simulink model "Sim_Runs_16p5"  (R2018b)
settings: Solver=FixedStepDiscrete  StartTime=0.0  StopTime=30  FixedStep=dt  RelTol=1e-3  EnableMultiTasking=on
PreLoadFcn:
  | DLLSimInit
InitFcn:
  | DLLSimInit
StartFcn:
  | tic
StopFcn:
  | SimTimeLaps = toc
values from neighbouring files (symbols this model uses):
  dt = 1/100    (= 0.01)    [DLLSimInit.m]    (also in DLLSimInit_SW.m; DLLSimInit_SW2.m; DLLSimInit_SW3.m)
  EngineLhFuelCut = 0    [DLLSimInit.m]    (also in DLLSimInit_SW.m; DLLSimInit_SW2.m; DLLSimInit_SW3.m)
  EngineRhFuelCut = 0    [DLLSimInit.m]    (also in DLLSimInit_SW.m; DLLSimInit_SW2.m; DLLSimInit_SW3.m)
  nDT = dt / SimDt    (= 6)    [DLLSimInit.m]    (also in DLLSimInit_SW.m; DLLSimInit_SW2.m; DLLSimInit_SW3.m)
  nOuputs = length(SaveList)    [DLLSimInit.m]    (also in DLLSimInit_SW.m; DLLSimInit_SW2.m; DLLSimInit_SW3.m)
  NWCastoring = 0    [DLLSimInit.m]
  PedalBrakeLh = 0    [DLLSimInit.m]    (also in DLLSimInit_SW.m; DLLSimInit_SW2.m; DLLSimInit_SW3.m)
  PedalBrakeRh = 0    [DLLSimInit.m]    (also in DLLSimInit_SW.m; DLLSimInit_SW2.m; DLLSimInit_SW3.m)
  RefWindDirDeg = WindDir    (= 90)    [DLLSimInit.m]    (also in DLLSimInit_SW.m; DLLSimInit_SW2.m; DLLSimInit_SW3.m)
  RefWindSpdKts = WindSpd    (= 0)    [DLLSimInit.m]    (also in DLLSimInit_SW.m; DLLSimInit_SW2.m; DLLSimInit_SW3.m)
  VertWindSpdKts = VertWindSpd    (= 0)    [DLLSimInit.m]
undefined symbols (not defined in the file or in its folder): DLLSimStep, sigbuilder_block, Trim_piccoloInCmd, Trim_REFSI_FD_IN_nmodeAftFlapCmd_Deg, Trim_REFSI_FD_IN_nmodeAilLhLowerCmd_Deg, Trim_REFSI_FD_IN_nmodeAilLhUpperCmd_Deg, Trim_REFSI_FD_IN_nmodeAilRhLowerCmd_Deg, Trim_REFSI_FD_IN_nmodeAilRhUpperCmd_Deg, Trim_REFSI_FD_IN_nmodeCgShifterCmd_Flag, Trim_REFSI_FD_IN_nmodeCgShifterCmd_Ft, Trim_REFSI_FD_IN_nmodeCgShifterNRCActive, Trim_REFSI_FD_IN_nmodeElvLhInbdCmd_Deg, Trim_REFSI_FD_IN_nmodeElvLhOutbdCmd_Deg, Trim_REFSI_FD_IN_nmodeElvLhUTailCmd_Deg, Trim_REFSI_FD_IN_nmodeElvRhInbdCmd_Deg, Trim_REFSI_FD_IN_nmodeElvRhOutbdCmd_Deg, Trim_REFSI_FD_IN_nmodeElvRhUTailCmd_Deg, Trim_REFSI_FD_IN_nmodeFlapLhIBCmd_Deg, Trim_REFSI_FD_IN_nmodeFlapLhOBCmd_Deg, Trim_REFSI_FD_IN_nmodeFlapRhIBCmd_Deg, Trim_REFSI_FD_IN_nmodeFlapRhOBCmd_Deg, Trim_REFSI_FD_IN_nmodeNoseGearCmd_Deg, Trim_REFSI_FD_IN_nmodeRudLhPylonCmd_Deg, Trim_REFSI_FD_IN_nmodeRudLhUTailCmd_Deg, Trim_REFSI_FD_IN_nmodeRudLhWingCmd_Deg, Trim_REFSI_FD_IN_nmodeRudRhPylonCmd_Deg, Trim_REFSI_FD_IN_nmodeRudRhUTailCmd_Deg, Trim_REFSI_FD_IN_nmodeRudRhWingCmd_Deg, Trim_REFSI_FD_IN_nmodeSlatLhCmd_Deg, Trim_REFSI_FD_IN_nmodeSlatRhCmd_Deg, Trim_REFSI_FD_IN_nmodeSplrLhInbdCmd_Deg, Trim_REFSI_FD_IN_nmodeSplrLhOutbdCmd_Deg, Trim_REFSI_FD_IN_nmodeSplrRhInbdCmd_Deg, Trim_REFSI_FD_IN_nmodeSplrRhOutbdCmd_Deg, Trim_REFSI_FD_IN_nmodeStabCmd, Trim_REFSI_FD_IN_nmodeTlaLhCmd_Deg, Trim_REFSI_FD_IN_nmodeTlaRhCmd_Deg
CloseFcn:
  | rtwprivate ssgencode ModelCloseRequest Sim_Runs
settings Model: ExtModeAutoUpdateStatusClock=off  Creator=b0514928  LastModifiedBy=B0532748
settings DataIOCC: LimitDataPoints=on  SaveFormat=Array  SaveState=on  SignalLogging=off
settings OptimizationCC: ExpressionDepthLimit=2147483647  LifeSpan=inf  SimCompilerOptimization=on
settings DebuggingCC: SaveWithParameterizedLinksMsg=none  UnderspecifiedInitializationDetection=Classic  MergeDetectMultiDrivingBlocksExec=none  SolverPrmCheckMsg=warning  StateNameClashWarn=warning  SFUnexpectedBacktrackingDiag=warning  SFNoUnconditionalDefaultTransitionDiag=warning  SFExecutionAtInitializationDiag=none
settings HardwareCC: ProdBitPerPointer=32  ProdBitPerSizeT=32  ProdBitPerPtrDiffT=32  ProdLargestAtomicFloat=None  ProdIntDivRoundTo=Undefined  ProdEndianess=Unspecified  ProdWordSize=32  ProdHWDeviceType=32-bit Generic
settings ModelReferenceCC: PropagateSignalLabelsOutOfModel=off
settings SFSimCC: SimUseLocalCustomCode=off
settings RTWCC: RTWUseLocalCustomCode=off
settings CodeAppCC: StateflowObjectComments=on
settings GRTTargetCC: TargetLangStandard=C89/C90 (ANSI)  GeneratePreprocessorConditionals=Disable all  CombineOutputUpdateFcns=off  GRTInterface=on
settings ConfigComp: CovMetricSettings=dw  CovHtmlReporting=on  CovSaveCumulativeToWorkspaceVar=on  CovSaveSingleToWorkspaceVar=on  CovExternalEMLEnable=off

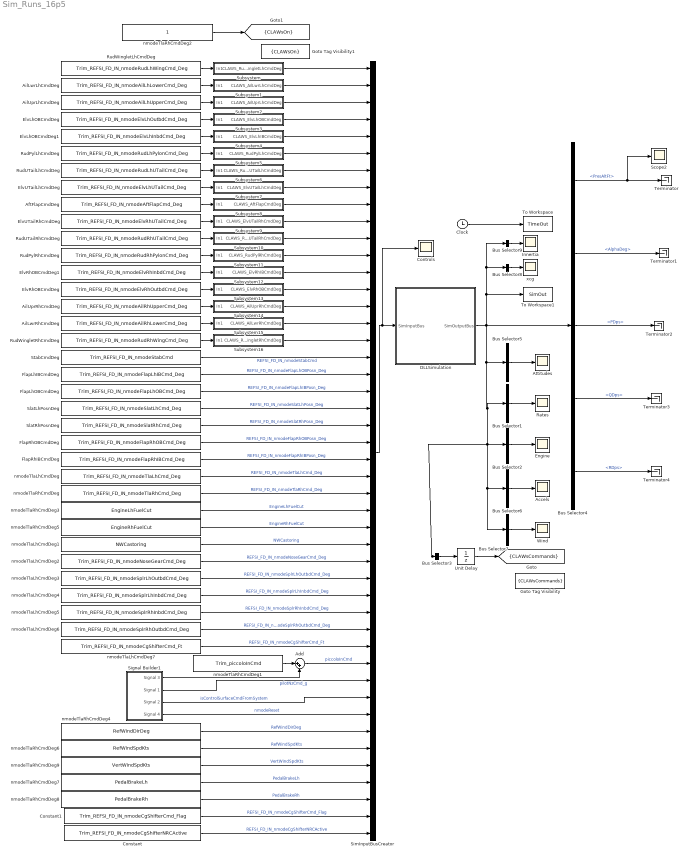
== system Sim_Runs_16p5 ==
  Accels : Scope
  Add : Sum  Inputs=|++
  AftFlapCmdDeg : Constant  Value=Trim_REFSI_FD_IN_nmodeAftFlapCmd_Deg
  AilLwrLhCmdDeg : Constant  Value=Trim_REFSI_FD_IN_nmodeAilLhLowerCmd_Deg
  AilLwrRhCmdDeg : Constant  Value=Trim_REFSI_FD_IN_nmodeAilRhLowerCmd_Deg
  AilUprLhCmdDeg : Constant  Value=Trim_REFSI_FD_IN_nmodeAilLhUpperCmd_Deg
  AilUprRhCmdDeg : Constant  Value=Trim_REFSI_FD_IN_nmodeAilRhUpperCmd_Deg
  Attitudes : Scope
  Bus Selector1 : BusSelector  OutputSignals=PDps,QDps,RDps  OutputAsBus=on
  Bus Selector2 : BusSelector  OutputSignals=XthrustLbs  OutputAsBus=on
  Bus Selector3 : BusSelector  OutputSignals=REFSI_AC_OUT_nmodeRudLhWingCmd_Deg,REFSI_AC_OUT_nmodeAilLhLowerCmd_Deg,REFSI_AC_OUT_nmodeAilLhUpperCmd_Deg,REFSI_AC_OUT_nmodeElvLhOutbdCmd_Deg,REFSI_AC_OUT_nmodeElvLhInbdCmd_Deg,REFSI_AC_OUT_nmodeRudLhPylonCmd_Deg,REFSI_AC_OUT_nmodeRudLhUTailCmd_Deg,REFSI_AC_OUT_nmodeElvLhUTailCmd_Deg,REFSI_AC_OUT_nmodeAftFlapCmd_Deg,REFSI_AC_OUT_nmodeElvRhUTailCmd_Deg,REFSI_AC_OUT_nmodeRudRhUTailCmd_Deg,REFSI_AC_OUT_nmodeRudRhPylonCmd_Deg,REFSI_AC_OUT_nmodeElvRhInbdCmd_Deg,REFSI_AC_OUT_nmodeElvRhOutbdCmd_Deg,REFSI_AC_OUT_nmodeAilRhUpperCmd_Deg,REFSI_AC_OUT_nmodeAilRhLowerCmd_Deg,REFSI_AC_OUT_nmodeRudRhWingCmd_Deg  OutputAsBus=on
  Bus Selector4 : BusSelector  OutputSignals=PresAltFt,AlphaDeg,PDps,QDps,RDps
  Bus Selector5 : BusSelector  OutputSignals=PhiDeg,ThetaDeg,PsiDeg  OutputAsBus=on
  Bus Selector6 : BusSelector  OutputSignals=NxG,NyG,NzG  OutputAsBus=on
  Bus Selector7 : BusSelector  OutputSignals=WindUFtps,WindVFtps,WindWFtps  OutputAsBus=on
  Bus Selector8 : BusSelector  OutputSignals=XcgPctMAC  OutputAsBus=on
  Bus Selector9 : BusSelector  OutputSignals=IxxLbsInch2,IyyLbsInch2,IzzLbsInch2,IxzLbsInch2  OutputAsBus=on
  Clock : Clock
  Constant : Constant  Value=Trim_REFSI_FD_IN_nmodeCgShifterNRCActive
  Constant1 : Constant  Value=Trim_REFSI_FD_IN_nmodeCgShifterCmd_Flag
  Controls : Scope
  DLLSimulation : Subsystem
  ElvLhOBCmdDeg : Constant  Value=Trim_REFSI_FD_IN_nmodeElvLhOutbdCmd_Deg
  ElvLhOBCmdDeg1 : Constant  Value=Trim_REFSI_FD_IN_nmodeElvLhInbdCmd_Deg
  ElvRhOBCmdDeg : Constant  Value=Trim_REFSI_FD_IN_nmodeElvRhOutbdCmd_Deg
  ElvRhOBCmdDeg1 : Constant  Value=Trim_REFSI_FD_IN_nmodeElvRhInbdCmd_Deg
  ElvUTailLhCmdDeg : Constant  Value=Trim_REFSI_FD_IN_nmodeElvLhUTailCmd_Deg
  ElvUTailRhCmdDeg : Constant  Value=Trim_REFSI_FD_IN_nmodeElvRhUTailCmd_Deg
  Engine : Scope
  FlapLhIBCmdDeg : Constant  Value=Trim_REFSI_FD_IN_nmodeFlapLhIBCmd_Deg
  FlapLhOBCmdDeg : Constant  Value=Trim_REFSI_FD_IN_nmodeFlapLhOBCmd_Deg
  FlapRhIBCmdDeg : Constant  Value=Trim_REFSI_FD_IN_nmodeFlapRhIBCmd_Deg
  FlapRhOBCmdDeg : Constant  Value=Trim_REFSI_FD_IN_nmodeFlapRhOBCmd_Deg
  Goto Tag Visibility : GotoTagVisibility  GotoTag=CLAWsCommands
  Goto Tag Visibility1 : GotoTagVisibility  GotoTag=CLAWsOn
  Innertia : Scope
  Rates : Scope
  RudPylLhCmdDeg : Constant  Value=Trim_REFSI_FD_IN_nmodeRudLhPylonCmd_Deg
  RudPylRhCmdDeg : Constant  Value=Trim_REFSI_FD_IN_nmodeRudRhPylonCmd_Deg
  RudUTailLhCmdDeg : Constant  Value=Trim_REFSI_FD_IN_nmodeRudLhUTailCmd_Deg
  RudUTailRhCmdDeg : Constant  Value=Trim_REFSI_FD_IN_nmodeRudRhUTailCmd_Deg
  RudWingletLhCmdDeg : Constant  Value=Trim_REFSI_FD_IN_nmodeRudLhWingCmd_Deg
  RudWingletRhCmdDeg : Constant  Value=Trim_REFSI_FD_IN_nmodeRudRhWingCmd_Deg
  Scope2 : Scope
  Signal Builder1 : Subsystem  Tag=STV Subsys  LoadFcn=sigbuilder_block('load');  StartFcn=sigbuilder_block('start');  StopFcn=sigbuilder_block('stop');  ClipboardFcn=sigbuilder_block('clipboard');  mask(Sigbuilder block){tuvar=[0:10]}
      mask help: Simulink:masks:SigbuilderBlock_MD
      mask init:
      | if ~strcmp(get_param(bdroot(gcbh),'SimulationStatus'),'stopped') tuvar = sigbuilder_block('maskInit'); end
      settings: CopyFcn=sigbuilder_block('copy');  DeleteFcn=sigbuilder_block('delete');  ModelCloseFcn=sigbuilder_block('modelClose');  PreSaveFcn=sigbuilder_block('preSave');  PauseFcn=sigbuilder_block('pause');  ContinueFcn=sigbuilder_block('continue');  NameChangeFcn=sigbuilder_block('namechange');  OpenFcn=sigbuilder_block('open',[703.5 198.75 550.5 360 ]);  CloseFcn=sigbuilder_block('close');
      mask Display: plot(0, 0, 100, 100,[2, 2, 32, 32, 2], [68, 8, 8, 68, 68],[32, 2], [38, 38], [32, 19, 2],[53, 60, 44], [32, 17, 17, 2],[16, 16, 31, 31]);txt = getActiveGroup(gcbh);text(2, 100, txt,'verticalAlignment', 'top');
  SimInputBusCreator : BusCreator  Inputs=46
  SlatLhPosnDeg : Constant  Value=Trim_REFSI_FD_IN_nmodeSlatLhCmd_Deg
  SlatRhPosnDeg : Constant  Value=Trim_REFSI_FD_IN_nmodeSlatRhCmd_Deg
  StabCmdDeg : Constant  Value=Trim_REFSI_FD_IN_nmodeStabCmd
  Subsystem : Subsystem
  Subsystem1 : Subsystem
  Subsystem10 : Subsystem
  Subsystem11 : Subsystem
  Subsystem12 : Subsystem
  Subsystem13 : Subsystem
  Subsystem14 : Subsystem
  Subsystem15 : Subsystem
  Subsystem16 : Subsystem
  Subsystem2 : Subsystem
  Subsystem3 : Subsystem
  Subsystem4 : Subsystem
  Subsystem5 : Subsystem
  Subsystem6 : Subsystem
  Subsystem7 : Subsystem
  Subsystem8 : Subsystem
  Subsystem9 : Subsystem
  Terminator{,1..4} (5 alike) : Terminator
  To Workspace : ToWorkspace  VariableName=TimeOut  SaveFormat=Structure With Time  SampleTime=-1
  To Workspace1 : ToWorkspace  VariableName=SimOut  SaveFormat=Structure With Time  SampleTime=-1
  Unit Delay : UnitDelay  SampleTime=-1
  Wind : Scope
  nmodeTlaLhCmdDeg : Constant  Value=Trim_REFSI_FD_IN_nmodeTlaLhCmd_Deg
  nmodeTlaLhCmdDeg1 : Constant  Value=NWCastoring
  nmodeTlaLhCmdDeg2 : Constant  Value=Trim_REFSI_FD_IN_nmodeNoseGearCmd_Deg
  nmodeTlaLhCmdDeg3 : Constant  Value=Trim_REFSI_FD_IN_nmodeSplrLhOutbdCmd_Deg
  nmodeTlaLhCmdDeg4 : Constant  Value=Trim_REFSI_FD_IN_nmodeSplrLhInbdCmd_Deg
  nmodeTlaLhCmdDeg5 : Constant  Value=Trim_REFSI_FD_IN_nmodeSplrRhInbdCmd_Deg
  nmodeTlaLhCmdDeg6 : Constant  Value=Trim_REFSI_FD_IN_nmodeSplrRhOutbdCmd_Deg
  nmodeTlaLhCmdDeg7 : Constant  Value=Trim_REFSI_FD_IN_nmodeCgShifterCmd_Ft
  nmodeTlaRhCmdDeg : Constant  Value=Trim_REFSI_FD_IN_nmodeTlaRhCmd_Deg
  nmodeTlaRhCmdDeg1 : Constant  Value=Trim_piccoloInCmd
  nmodeTlaRhCmdDeg2 : Constant
  nmodeTlaRhCmdDeg3 : Constant  Value=EngineLhFuelCut
  nmodeTlaRhCmdDeg4 : Constant  Value=RefWindDirDeg
  nmodeTlaRhCmdDeg5 : Constant  Value=EngineRhFuelCut
  nmodeTlaRhCmdDeg6 : Constant  Value=RefWindSpdKts
  nmodeTlaRhCmdDeg7 : Constant  Value=PedalBrakeLh
  nmodeTlaRhCmdDeg8 : Constant  Value=PedalBrakeRh
  nmodeTlaRhCmdDeg9 : Constant  Value=VertWindSpdKts
  xcg : Scope
  tag scope: CLAWsCommands=scoped, CLAWsOn=scoped
  wires:
  Clock/1 -> To Workspace/1
  SimInputBusCreator/1 -> Controls/1, DLLSimulation/1(SimInputBus)
  Bus Selector4/1 -> Scope2/1, Terminator/1  "<PresAltFt>"
  Bus Selector4/2 -> Terminator1/1  "<AlphaDeg>"
  Bus Selector4/3 -> Terminator2/1  "<PDps>"
  Bus Selector4/4 -> Terminator3/1  "<QDps>"
  Bus Selector4/5 -> Terminator4/1  "<RDps>"
  AilLwrLhCmdDeg/1 -> Subsystem1/1(In1)
  AilUprLhCmdDeg/1 -> Subsystem2/1(In1)
  ElvLhOBCmdDeg/1 -> Subsystem3/1(In1)
  RudPylLhCmdDeg/1 -> Subsystem5/1(In1)
  RudUTailLhCmdDeg/1 -> Subsystem6/1(In1)
  ElvUTailLhCmdDeg/1 -> Subsystem7/1(In1)
  AftFlapCmdDeg/1 -> Subsystem8/1(In1)
  ElvUTailRhCmdDeg/1 -> Subsystem9/1(In1)
  RudUTailRhCmdDeg/1 -> Subsystem10/1(In1)
  RudPylRhCmdDeg/1 -> Subsystem11/1(In1)
  ElvRhOBCmdDeg/1 -> Subsystem13/1(In1)
  AilUprRhCmdDeg/1 -> Subsystem14/1(In1)
  AilLwrRhCmdDeg/1 -> Subsystem15/1(In1)
  RudWingletRhCmdDeg/1 -> Subsystem16/1(In1)
  StabCmdDeg/1 -> SimInputBusCreator/18  "REFSI_FD_IN_nmodeStabCmd"
  FlapLhIBCmdDeg/1 -> SimInputBusCreator/19  "REFSI_FD_IN_nmodeFlapLhOBPosn_Deg"
  FlapLhOBCmdDeg/1 -> SimInputBusCreator/20  "REFSI_FD_IN_nmodeFlapLhIBPosn_Deg"
  SlatLhPosnDeg/1 -> SimInputBusCreator/21  "REFSI_FD_IN_nmodeSlatLhPosn_Deg"
  SlatRhPosnDeg/1 -> SimInputBusCreator/22  "REFSI_FD_IN_nmodeSlatRhPosn_Deg"
  FlapRhOBCmdDeg/1 -> SimInputBusCreator/23  "REFSI_FD_IN_nmodeFlapRhOBPosn_Deg"
  FlapRhIBCmdDeg/1 -> SimInputBusCreator/24  "REFSI_FD_IN_nmodeFlapRhIBPosn_Deg"
  nmodeTlaLhCmdDeg/1 -> SimInputBusCreator/25  "REFSI_FD_IN_nmodeTlaLhCmd_Deg"
  nmodeTlaRhCmdDeg/1 -> SimInputBusCreator/26  "REFSI_FD_IN_nmodeTlaRhCmd_Deg"
  Bus Selector2/1 -> Engine/1
  Bus Selector1/1 -> Rates/1
  DLLSimulation/1(SimOutputBus) -> Bus Selector4/1, Bus Selector9/1, Bus Selector8/1, To Workspace1/1, Bus Selector5/1, Bus Selector7/1, Bus Selector6/1, Bus Selector3/1, Bus Selector2/1, Bus Selector1/1
  ElvLhOBCmdDeg1/1 -> Subsystem4/1(In1)
  ElvRhOBCmdDeg1/1 -> Subsystem12/1(In1)
  Bus Selector3/1 -> Unit Delay/1
  RudWingletLhCmdDeg/1 -> Subsystem/1(In1)
  Subsystem/1(CLAWS_RudWingletLhCmdDeg) -> SimInputBusCreator/1
  Subsystem1/1(CLAWS_AilLwrLhCmdDeg) -> SimInputBusCreator/2
  Subsystem2/1(CLAWS_AilUprLhCmdDeg) -> SimInputBusCreator/3
  Subsystem3/1(CLAWS_ElvLhOBCmdDeg) -> SimInputBusCreator/4
  Subsystem4/1(CLAWS_ElvLhIBCmdDeg) -> SimInputBusCreator/5
  Subsystem5/1(CLAWS_RudPylLhCmdDeg) -> SimInputBusCreator/6
  Subsystem6/1(CLAWS_RudUTailLhCmdDeg) -> SimInputBusCreator/7
  Subsystem7/1(CLAWS_ElvUTailLhCmdDeg) -> SimInputBusCreator/8
  Subsystem8/1(CLAWS_AftFlapCmdDeg) -> SimInputBusCreator/9
  Subsystem9/1(CLAWS_ElvUTailRhCmdDeg) -> SimInputBusCreator/10
  Subsystem10/1(CLAWS_RudUTailRhCmdDeg) -> SimInputBusCreator/11
  Subsystem11/1(CLAWS_RudPylRhCmdDeg) -> SimInputBusCreator/12
  Subsystem12/1(CLAWS_ElvRhIBCmdDeg) -> SimInputBusCreator/13
  Subsystem13/1(CLAWS_ElvRhOBCmdDeg) -> SimInputBusCreator/14
  Subsystem14/1(CLAWS_AilUprRhCmdDeg) -> SimInputBusCreator/15
  Subsystem15/1(CLAWS_AilLwrRhCmdDeg) -> SimInputBusCreator/16
  Subsystem16/1(CLAWS_RudWingletRhCmdDeg) -> SimInputBusCreator/17
  nmodeTlaRhCmdDeg2/1 -> [CLAWsOn]
  Unit Delay/1 -> [CLAWsCommands]
  nmodeTlaRhCmdDeg1/1 -> Add/1
  Add/1 -> SimInputBusCreator/36  "piccoloInCmd"
  Signal Builder1/1(Signal 3) -> Add/2
  Signal Builder1/2(Signal 1) -> SimInputBusCreator/37  "pilotNzCmd_g"
  Signal Builder1/3(Signal 2) -> SimInputBusCreator/38  "isControlSurfaceCmdFromSystem"
  Signal Builder1/4(Signal 4) -> SimInputBusCreator/39  "nmodeReset"
  Bus Selector5/1 -> Attitudes/1
  Bus Selector6/1 -> Accels/1
  nmodeTlaLhCmdDeg2/1 -> SimInputBusCreator/30  "REFSI_FD_IN_nmodeNoseGearCmd_Deg"
  Bus Selector8/1 -> xcg/1
  Bus Selector9/1 -> Innertia/1
  Bus Selector7/1 -> Wind/1
  nmodeTlaLhCmdDeg3/1 -> SimInputBusCreator/31  "REFSI_FD_IN_nmodeSplrLhOutbdCmd_Deg"
  nmodeTlaLhCmdDeg4/1 -> SimInputBusCreator/32  "REFSI_FD_IN_nmodeSplrLhInbdCmd_Deg"
  nmodeTlaLhCmdDeg5/1 -> SimInputBusCreator/33  "REFSI_FD_IN_nmodeSplrRhInbdCmd_Deg"
  nmodeTlaLhCmdDeg6/1 -> SimInputBusCreator/34  "REFSI_FD_IN_nmodeSplrRhOutbdCmd_Deg"
  nmodeTlaLhCmdDeg7/1 -> SimInputBusCreator/35  "REFSI_FD_IN_nmodeCgShifterCmd_Ft"
  nmodeTlaLhCmdDeg1/1 -> SimInputBusCreator/29  "NWCastoring"
  nmodeTlaRhCmdDeg3/1 -> SimInputBusCreator/27  "EngineLhFuelCut"
  nmodeTlaRhCmdDeg5/1 -> SimInputBusCreator/28  "EngineRhFuelCut"
  nmodeTlaRhCmdDeg4/1 -> SimInputBusCreator/40  "RefWindDirDeg"
  nmodeTlaRhCmdDeg6/1 -> SimInputBusCreator/41  "RefWindSpdKts"
  nmodeTlaRhCmdDeg7/1 -> SimInputBusCreator/43  "PedalBrakeLh"
  nmodeTlaRhCmdDeg8/1 -> SimInputBusCreator/44  "PedalBrakeRh"
  nmodeTlaRhCmdDeg9/1 -> SimInputBusCreator/42  "VertWindSpdKts"
  Constant1/1 -> SimInputBusCreator/45  "REFSI_FD_IN_nmodeCgShifterCmd_Flag"
  Constant/1 -> SimInputBusCreator/46  "REFSI_FD_IN_nmodeCgShifterNRCActive"

== system Sim_Runs_16p5/DLLSimulation ==
  SimInputBus : Inport
  Bus2Vect2 : Subsystem
      mask init:
      | CurrentSys = gcs;
      | blockName = get_param(gcb,'Name');
      | 
      | CurBlk = [CurrentSys,'/',blockName];%Current block
      | BusSel = [CurrentSys,'/',blockName,'/BusSelector'];%BusSelectorBlock
      | BusMux = [CurrentSys,'/',blockName,'/Mux'];%Mux bloxk
      | 
      | 
      | 
      | Inputs = get_param(BusSel,'InputSignals');
      | 
      | 
      | outsig='';
      | for i=1:length(Inputs)
      |     outsig=[outsig Inputs{i} ','];
      | end;
      | outsig=outsig(1:length(outsig)-1);
      | 
      |     for nnn = 1:str2double(get_param(BusMux,'Inputs'))
      |         delete_line([CurrentSys '/' blockName],['BusSelector/' num2str(nnn)],['Mux/' num2str(nnn)])
      |     end
      |     
      | set_param(BusSel,'OutputSignals',outsig);
      | set_param(BusMux,'Inputs',num2str(length(Inputs)))
      | 
      | 
      | 
      |     
      |     for nnn = 1:length(Inputs)
      |         add_line([CurrentSys '/' blockName],['BusSelector/' num2str(nnn)],['Mux/' num2str(nnn)])
      |     end
  DLLSimulationStep : MATLABFcn  MATLABFcn=DLLSimStep(u,nDT)  OutputDimensions=nOuputs  SampleTime=dt
  Vector to Bus : Subsystem  mask{Nsigs=nOuputs}
      mask prompts: Nsigs "Signal Length"
  SimOutputBus : Outport
  wires:
  Bus2Vect2/1(Out1) -> DLLSimulationStep/1
  DLLSimulationStep/1 -> Vector to Bus/1(In1)
  Vector to Bus/1(Out1) -> SimOutputBus/1
  SimInputBus/1 -> Bus2Vect2/1(In1)

== system Sim_Runs_16p5/Signal Builder1 ==
  Demux : Demux  Tag=STV Demux
  FromWs : FromWorkspace  Tag=STV FromWs  VariableName=tuvar  SampleTime=0
      SigBuilderData=|
      | common.afterFinalStr = 'Extrapolate'
      | common.sampleTime = 0
      | dataSet.timeRange = [0 50]
      | dataSet.name = 'Group 1'
      | sbobj.Groups.Name = 'Group 1'
      | sbobj.Groups.Signals(1).Name = 'Signal 3'
      | sbobj.Groups.Signals(1).XData = [0 1 1 50]
      | sbobj.Groups.Signals(1).YData = [0 0 -1 -1]
      | sbobj.Groups.Signals(2).Name = 'Signal 1'
      | sbobj.Groups.Signals(2).XData = [0 20 20 30 30 50]
      | sbobj.Groups.Signals(2).YData = [0 0 0.4 0.4 0 0]
      | sbobj.Groups.Signals(3).Name = 'Signal 2'
      | sbobj.Groups.Signals(3).XData = [0 0.5 0.5 50]
      | sbobj.Groups.Signals(3).YData = [1 1 0 0]
      | sbobj.Groups.Signals(4).Name = 'Signal 4'
      | sbobj.Groups.Signals(4).XData = [0 0.1 0.1 50]
      | sbobj.Groups.Signals(4).YData = [1 1 0 0]
      | sbobj.Groups.TimeRange = [0 50]
  Signal 3 : Outport  Tag=STV Outport
  Signal 1 : Outport  Tag=STV Outport  Port=2
  Signal 2 : Outport  Tag=STV Outport  Port=3
  Signal 4 : Outport  Tag=STV Outport  Port=4
  wires:
  FromWs/1 -> Demux/1
  Demux/1 -> Signal 3/1
  Demux/2 -> Signal 1/1
  Demux/3 -> Signal 2/1
  Demux/4 -> Signal 4/1

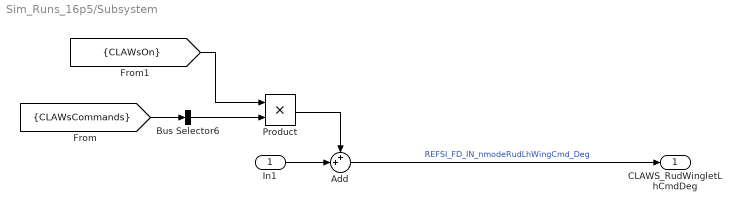
== system Sim_Runs_16p5/Subsystem ==
  In1 : Inport
  Add : Sum  Inputs=++|
  Bus Selector6 : BusSelector  OutputSignals=REFSI_AC_OUT_nmodeRudLhWingCmd_Deg  OutputAsBus=on
  Product : Product
  CLAWS_RudWingletLhCmdDeg : Outport
  wires:
  Add/1 -> CLAWS_RudWingletLhCmdDeg/1  "REFSI_FD_IN_nmodeRudLhWingCmd_Deg"
  [CLAWsCommands] -> Bus Selector6/1
  In1/1 -> Add/2
  Bus Selector6/1 -> Product/2
  Product/1 -> Add/1
  [CLAWsOn] -> Product/1

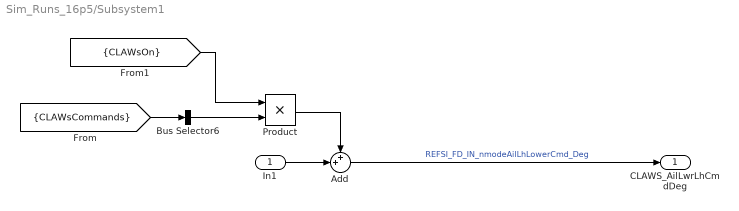
== system Sim_Runs_16p5/Subsystem1 ==
  In1 : Inport
  Add : Sum  Inputs=++|
  Bus Selector6 : BusSelector  OutputSignals=REFSI_AC_OUT_nmodeAilLhLowerCmd_Deg  OutputAsBus=on
  Product : Product
  CLAWS_AilLwrLhCmdDeg : Outport
  wires:
  [CLAWsOn] -> Product/1
  Product/1 -> Add/1
  Bus Selector6/1 -> Product/2
  In1/1 -> Add/2
  [CLAWsCommands] -> Bus Selector6/1
  Add/1 -> CLAWS_AilLwrLhCmdDeg/1  "REFSI_FD_IN_nmodeAilLhLowerCmd_Deg"

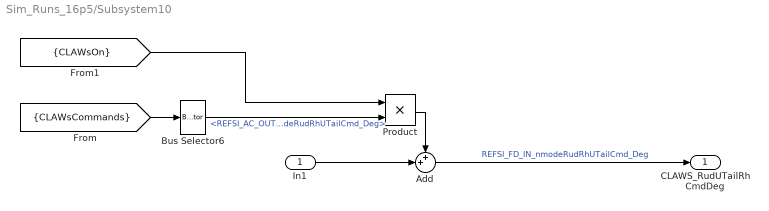
== system Sim_Runs_16p5/Subsystem10 ==
  In1 : Inport
  Add : Sum  Inputs=++|
  Bus Selector6 : BusSelector  OutputSignals=REFSI_AC_OUT_nmodeRudRhUTailCmd_Deg
  Product : Product
  CLAWS_RudUTailRhCmdDeg : Outport
  wires:
  Add/1 -> CLAWS_RudUTailRhCmdDeg/1  "REFSI_FD_IN_nmodeRudRhUTailCmd_Deg"
  [CLAWsCommands] -> Bus Selector6/1
  In1/1 -> Add/2
  Bus Selector6/1 -> Product/2  "<REFSI_AC_OUT_nmodeRudRhUTailCmd_Deg>"
  Product/1 -> Add/1
  [CLAWsOn] -> Product/1

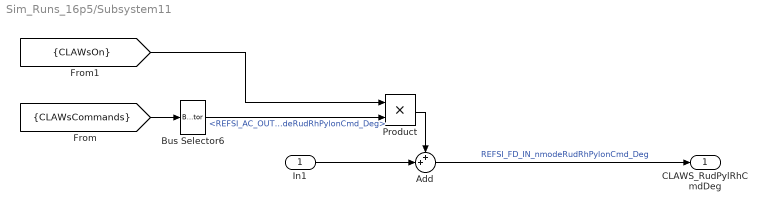
== system Sim_Runs_16p5/Subsystem11 ==
  In1 : Inport
  Add : Sum  Inputs=++|
  Bus Selector6 : BusSelector  OutputSignals=REFSI_AC_OUT_nmodeRudRhPylonCmd_Deg
  Product : Product
  CLAWS_RudPylRhCmdDeg : Outport
  wires:
  [CLAWsOn] -> Product/1
  Product/1 -> Add/1
  Bus Selector6/1 -> Product/2  "<REFSI_AC_OUT_nmodeRudRhPylonCmd_Deg>"
  In1/1 -> Add/2
  [CLAWsCommands] -> Bus Selector6/1
  Add/1 -> CLAWS_RudPylRhCmdDeg/1  "REFSI_FD_IN_nmodeRudRhPylonCmd_Deg"

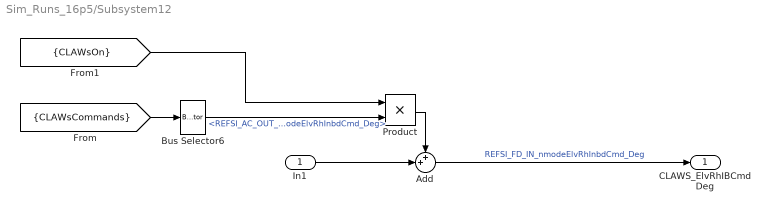
== system Sim_Runs_16p5/Subsystem12 ==
  In1 : Inport
  Add : Sum  Inputs=++|
  Bus Selector6 : BusSelector  OutputSignals=REFSI_AC_OUT_nmodeElvRhInbdCmd_Deg
  Product : Product
  CLAWS_ElvRhIBCmdDeg : Outport
  wires:
  Add/1 -> CLAWS_ElvRhIBCmdDeg/1  "REFSI_FD_IN_nmodeElvRhInbdCmd_Deg"
  [CLAWsCommands] -> Bus Selector6/1
  In1/1 -> Add/2
  Bus Selector6/1 -> Product/2  "<REFSI_AC_OUT_nmodeElvRhInbdCmd_Deg>"
  Product/1 -> Add/1
  [CLAWsOn] -> Product/1

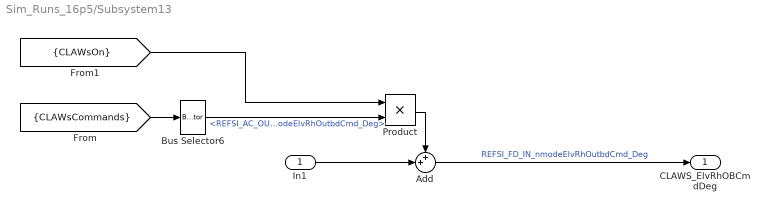
== system Sim_Runs_16p5/Subsystem13 ==
  In1 : Inport
  Add : Sum  Inputs=++|
  Bus Selector6 : BusSelector  OutputSignals=REFSI_AC_OUT_nmodeElvRhOutbdCmd_Deg
  Product : Product
  CLAWS_ElvRhOBCmdDeg : Outport
  wires:
  [CLAWsOn] -> Product/1
  Product/1 -> Add/1
  Bus Selector6/1 -> Product/2  "<REFSI_AC_OUT_nmodeElvRhOutbdCmd_Deg>"
  In1/1 -> Add/2
  [CLAWsCommands] -> Bus Selector6/1
  Add/1 -> CLAWS_ElvRhOBCmdDeg/1  "REFSI_FD_IN_nmodeElvRhOutbdCmd_Deg"

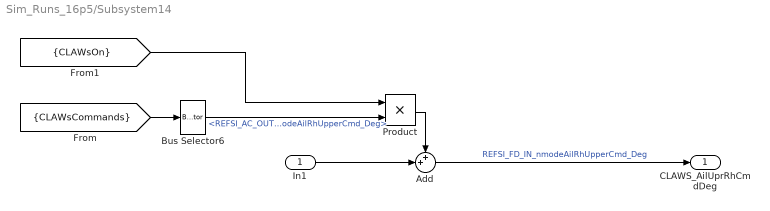
== system Sim_Runs_16p5/Subsystem14 ==
  In1 : Inport
  Add : Sum  Inputs=++|
  Bus Selector6 : BusSelector  OutputSignals=REFSI_AC_OUT_nmodeAilRhUpperCmd_Deg
  Product : Product
  CLAWS_AilUprRhCmdDeg : Outport
  wires:
  Add/1 -> CLAWS_AilUprRhCmdDeg/1  "REFSI_FD_IN_nmodeAilRhUpperCmd_Deg"
  [CLAWsCommands] -> Bus Selector6/1
  In1/1 -> Add/2
  Bus Selector6/1 -> Product/2  "<REFSI_AC_OUT_nmodeAilRhUpperCmd_Deg>"
  Product/1 -> Add/1
  [CLAWsOn] -> Product/1

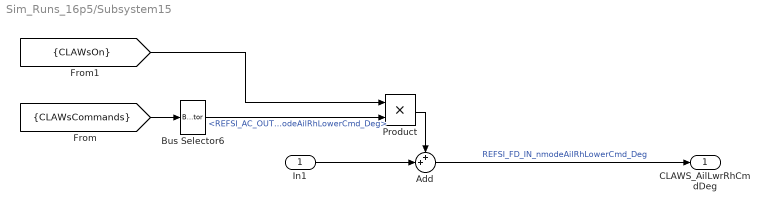
== system Sim_Runs_16p5/Subsystem15 ==
  In1 : Inport
  Add : Sum  Inputs=++|
  Bus Selector6 : BusSelector  OutputSignals=REFSI_AC_OUT_nmodeAilRhLowerCmd_Deg
  Product : Product
  CLAWS_AilLwrRhCmdDeg : Outport
  wires:
  [CLAWsOn] -> Product/1
  Product/1 -> Add/1
  Bus Selector6/1 -> Product/2  "<REFSI_AC_OUT_nmodeAilRhLowerCmd_Deg>"
  In1/1 -> Add/2
  [CLAWsCommands] -> Bus Selector6/1
  Add/1 -> CLAWS_AilLwrRhCmdDeg/1  "REFSI_FD_IN_nmodeAilRhLowerCmd_Deg"

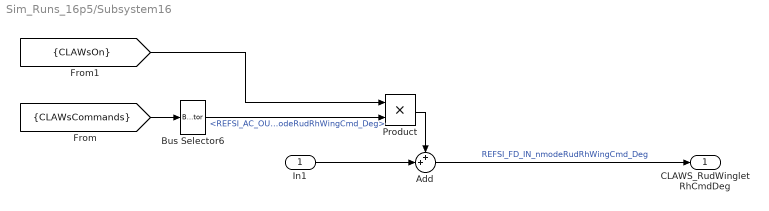
== system Sim_Runs_16p5/Subsystem16 ==
  In1 : Inport
  Add : Sum  Inputs=++|
  Bus Selector6 : BusSelector  OutputSignals=REFSI_AC_OUT_nmodeRudRhWingCmd_Deg
  Product : Product
  CLAWS_RudWingletRhCmdDeg : Outport
  wires:
  Add/1 -> CLAWS_RudWingletRhCmdDeg/1  "REFSI_FD_IN_nmodeRudRhWingCmd_Deg"
  [CLAWsCommands] -> Bus Selector6/1
  In1/1 -> Add/2
  Bus Selector6/1 -> Product/2  "<REFSI_AC_OUT_nmodeRudRhWingCmd_Deg>"
  Product/1 -> Add/1
  [CLAWsOn] -> Product/1

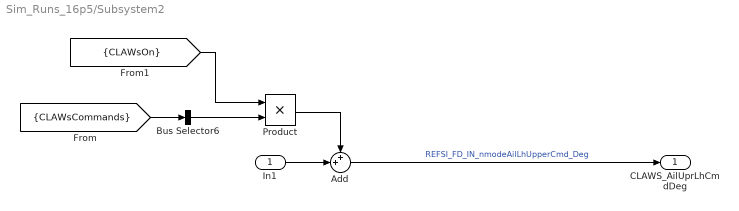
== system Sim_Runs_16p5/Subsystem2 ==
  In1 : Inport
  Add : Sum  Inputs=++|
  Bus Selector6 : BusSelector  OutputSignals=REFSI_AC_OUT_nmodeAilLhUpperCmd_Deg  OutputAsBus=on
  Product : Product
  CLAWS_AilUprLhCmdDeg : Outport
  wires:
  Add/1 -> CLAWS_AilUprLhCmdDeg/1  "REFSI_FD_IN_nmodeAilLhUpperCmd_Deg"
  [CLAWsCommands] -> Bus Selector6/1
  In1/1 -> Add/2
  Bus Selector6/1 -> Product/2
  Product/1 -> Add/1
  [CLAWsOn] -> Product/1

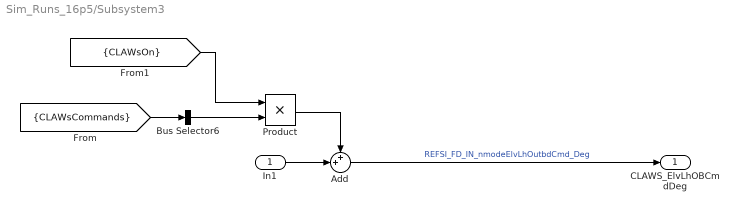
== system Sim_Runs_16p5/Subsystem3 ==
  In1 : Inport
  Add : Sum  Inputs=++|
  Bus Selector6 : BusSelector  OutputSignals=REFSI_AC_OUT_nmodeElvLhOutbdCmd_Deg  OutputAsBus=on
  Product : Product
  CLAWS_ElvLhOBCmdDeg : Outport
  wires:
  [CLAWsOn] -> Product/1
  Product/1 -> Add/1
  Bus Selector6/1 -> Product/2
  In1/1 -> Add/2
  [CLAWsCommands] -> Bus Selector6/1
  Add/1 -> CLAWS_ElvLhOBCmdDeg/1  "REFSI_FD_IN_nmodeElvLhOutbdCmd_Deg"

== system Sim_Runs_16p5/Subsystem4 ==
  In1 : Inport
  Add : Sum  Inputs=++|
  Bus Selector6 : BusSelector  OutputSignals=REFSI_AC_OUT_nmodeElvLhInbdCmd_Deg  OutputAsBus=on
  Product : Product
  CLAWS_ElvLhIBCmdDeg : Outport
  wires:
  Add/1 -> CLAWS_ElvLhIBCmdDeg/1  "REFSI_FD_IN_nmodeElvLhInbdCmd_Deg"
  [CLAWsCommands] -> Bus Selector6/1
  In1/1 -> Add/2
  Bus Selector6/1 -> Product/2
  Product/1 -> Add/1
  [CLAWsOn] -> Product/1

== system Sim_Runs_16p5/Subsystem5 ==
  In1 : Inport
  Add : Sum  Inputs=++|
  Bus Selector6 : BusSelector  OutputSignals=REFSI_AC_OUT_nmodeRudLhPylonCmd_Deg
  Product : Product
  CLAWS_RudPylLhCmdDeg : Outport
  wires:
  [CLAWsOn] -> Product/1
  Product/1 -> Add/1
  Bus Selector6/1 -> Product/2  "<REFSI_AC_OUT_nmodeRudLhPylonCmd_Deg>"
  In1/1 -> Add/2
  [CLAWsCommands] -> Bus Selector6/1
  Add/1 -> CLAWS_RudPylLhCmdDeg/1  "REFSI_FD_IN_nmodeRudLhPylonCmd_Deg"

== system Sim_Runs_16p5/Subsystem6 ==
  In1 : Inport
  Add : Sum  Inputs=++|
  Bus Selector6 : BusSelector  OutputSignals=REFSI_AC_OUT_nmodeRudLhUTailCmd_Deg
  Product : Product
  CLAWS_RudUTailLhCmdDeg : Outport
  wires:
  Add/1 -> CLAWS_RudUTailLhCmdDeg/1  "REFSI_FD_IN_nmodeRudLhUTailCmd_Deg"
  [CLAWsCommands] -> Bus Selector6/1
  In1/1 -> Add/2
  Bus Selector6/1 -> Product/2  "<REFSI_AC_OUT_nmodeRudLhUTailCmd_Deg>"
  Product/1 -> Add/1
  [CLAWsOn] -> Product/1

== system Sim_Runs_16p5/Subsystem7 ==
  In1 : Inport
  Add : Sum  Inputs=++|
  Bus Selector6 : BusSelector  OutputSignals=REFSI_AC_OUT_nmodeElvLhUTailCmd_Deg
  Product : Product
  CLAWS_ElvUTailLhCmdDeg : Outport
  wires:
  [CLAWsOn] -> Product/1
  Product/1 -> Add/1
  Bus Selector6/1 -> Product/2  "<REFSI_AC_OUT_nmodeElvLhUTailCmd_Deg>"
  In1/1 -> Add/2
  [CLAWsCommands] -> Bus Selector6/1
  Add/1 -> CLAWS_ElvUTailLhCmdDeg/1  "REFSI_FD_IN_nmodeElvLhUTailCmd_Deg"

== system Sim_Runs_16p5/Subsystem8 ==
  In1 : Inport
  Add : Sum  Inputs=++|
  Bus Selector6 : BusSelector  OutputSignals=REFSI_AC_OUT_nmodeAftFlapCmd_Deg
  Product : Product
  CLAWS_AftFlapCmdDeg : Outport
  wires:
  Add/1 -> CLAWS_AftFlapCmdDeg/1  "REFSI_FD_IN_nmodeAftFlapCmd_Deg"
  [CLAWsCommands] -> Bus Selector6/1
  In1/1 -> Add/2
  Bus Selector6/1 -> Product/2  "<REFSI_AC_OUT_nmodeAftFlapCmd_Deg>"
  Product/1 -> Add/1
  [CLAWsOn] -> Product/1

== system Sim_Runs_16p5/Subsystem9 ==
  In1 : Inport
  Add : Sum  Inputs=++|
  Bus Selector6 : BusSelector  OutputSignals=REFSI_AC_OUT_nmodeElvRhUTailCmd_Deg
  Product : Product
  CLAWS_ElvUTailRhCmdDeg : Outport
  wires:
  [CLAWsOn] -> Product/1
  Product/1 -> Add/1
  Bus Selector6/1 -> Product/2  "<REFSI_AC_OUT_nmodeElvRhUTailCmd_Deg>"
  In1/1 -> Add/2
  [CLAWsCommands] -> Bus Selector6/1
  Add/1 -> CLAWS_ElvUTailRhCmdDeg/1  "REFSI_FD_IN_nmodeElvRhUTailCmd_Deg"

== system Sim_Runs_16p5/DLLSimulation/Bus2Vect2 ==
  In1 : Inport
  BusSelector : BusSelector  OutputSignals=REFSI_FD_IN_nmodeRudLhWingCmd_Deg,REFSI_FD_IN_nmodeAilLhLowerCmd_Deg,REFSI_FD_IN_nmodeAilLhUpperCmd_Deg,REFSI_FD_IN_nmodeElvLhOutbdCmd_Deg,REFSI_FD_IN_nmodeElvLhInbdCmd_Deg,REFSI_FD_IN_nmodeRudLhPylonCmd_Deg,REFSI_FD_IN_nmodeRudLhUTailCmd_Deg,REFSI_FD_IN_nmodeElvLhUTailCmd_Deg,REFSI_FD_IN_nmodeAftFlapCmd_Deg,REFSI_FD_IN_nmodeElvRhUTailCmd_Deg,REFSI_FD_IN_nmodeRudRhUTailCmd_Deg,REFSI_FD_IN_nmodeRudRhPylonCmd_Deg,REFSI_FD_IN_nmodeElvRhInbdCmd_Deg,REFSI_FD_IN_nmodeElvRhOutbdCmd_Deg,REFSI_FD_IN_nmodeAilRhUpperCmd_Deg,REFSI_FD_IN_nmodeAilRhLowerCmd_Deg,REFSI_FD_IN_nmodeRudRhWingCmd_Deg,REFSI_FD_IN_nmodeStabCmd,REFSI_FD_IN_nmodeFlapLhOBPosn_Deg,REFSI_FD_IN_nmodeFlapLhIBPosn_Deg,REFSI_FD_IN_nmodeSlatLhPosn_Deg,REFSI_FD_IN_nmodeSlatRhPosn_Deg,REFSI_FD_IN_nmodeFlapRhOBPosn_Deg,REFSI_FD_IN_nmodeFlapRhIBPosn_Deg,REFSI_FD_IN_nmodeTlaLhCmd_Deg,REFSI_FD_IN_nmodeTlaRhCmd_Deg,EngineLhFuelCut,EngineRhFuelCut,NWCastoring,REFSI_FD_IN_nmodeNoseGearCmd_Deg,REFSI_FD_IN_nmodeSplrLhOutbdCmd_Deg,REFSI_FD_IN_nmodeSplrLhInbdCmd_Deg,REFSI_FD_IN_nmodeSplrRhInbdCmd_Deg,REFSI_FD_IN_nmodeSplrRhOutbdCmd_Deg,REFSI_FD_IN_nmodeCgShifterCmd_Ft,piccoloInCmd,pilotNzCmd_g,isControlSurfaceCmdFromSystem,nmodeReset,RefWindDirDeg,RefWindSpdKts,VertWindSpdKts,PedalBrakeLh,PedalBrakeRh,REFSI_FD_IN_nmodeCgShifterCmd_Flag,REFSI_FD_IN_nmodeCgShifterNRCActive
  Mux : Mux  Inputs=46
  Out1 : Outport
  wires:
  In1/1 -> BusSelector/1
  Mux/1 -> Out1/1
  BusSelector/1 -> Mux/1  "<REFSI_FD_IN_nmodeRudLhWingCmd_Deg>"
  BusSelector/2 -> Mux/2  "<REFSI_FD_IN_nmodeAilLhLowerCmd_Deg>"
  BusSelector/3 -> Mux/3  "<REFSI_FD_IN_nmodeAilLhUpperCmd_Deg>"
  BusSelector/4 -> Mux/4  "<REFSI_FD_IN_nmodeElvLhOutbdCmd_Deg>"
  BusSelector/5 -> Mux/5  "<REFSI_FD_IN_nmodeElvLhInbdCmd_Deg>"
  BusSelector/6 -> Mux/6  "<REFSI_FD_IN_nmodeRudLhPylonCmd_Deg>"
  BusSelector/7 -> Mux/7  "<REFSI_FD_IN_nmodeRudLhUTailCmd_Deg>"
  BusSelector/8 -> Mux/8  "<REFSI_FD_IN_nmodeElvLhUTailCmd_Deg>"
  BusSelector/9 -> Mux/9  "<REFSI_FD_IN_nmodeAftFlapCmd_Deg>"
  BusSelector/10 -> Mux/10  "<REFSI_FD_IN_nmodeElvRhUTailCmd_Deg>"
  BusSelector/11 -> Mux/11  "<REFSI_FD_IN_nmodeRudRhUTailCmd_Deg>"
  BusSelector/12 -> Mux/12  "<REFSI_FD_IN_nmodeRudRhPylonCmd_Deg>"
  BusSelector/13 -> Mux/13  "<REFSI_FD_IN_nmodeElvRhInbdCmd_Deg>"
  BusSelector/14 -> Mux/14  "<REFSI_FD_IN_nmodeElvRhOutbdCmd_Deg>"
  BusSelector/15 -> Mux/15  "<REFSI_FD_IN_nmodeAilRhUpperCmd_Deg>"
  BusSelector/16 -> Mux/16  "<REFSI_FD_IN_nmodeAilRhLowerCmd_Deg>"
  BusSelector/17 -> Mux/17  "<REFSI_FD_IN_nmodeRudRhWingCmd_Deg>"
  BusSelector/18 -> Mux/18  "<REFSI_FD_IN_nmodeStabCmd>"
  BusSelector/19 -> Mux/19  "<REFSI_FD_IN_nmodeFlapLhOBPosn_Deg>"
  BusSelector/20 -> Mux/20  "<REFSI_FD_IN_nmodeFlapLhIBPosn_Deg>"
  BusSelector/21 -> Mux/21  "<REFSI_FD_IN_nmodeSlatLhPosn_Deg>"
  BusSelector/22 -> Mux/22  "<REFSI_FD_IN_nmodeSlatRhPosn_Deg>"
  BusSelector/23 -> Mux/23  "<REFSI_FD_IN_nmodeFlapRhOBPosn_Deg>"
  BusSelector/24 -> Mux/24  "<REFSI_FD_IN_nmodeFlapRhIBPosn_Deg>"
  BusSelector/25 -> Mux/25  "<REFSI_FD_IN_nmodeTlaLhCmd_Deg>"
  BusSelector/26 -> Mux/26  "<REFSI_FD_IN_nmodeTlaRhCmd_Deg>"
  BusSelector/27 -> Mux/27  "<EngineLhFuelCut>"
  BusSelector/28 -> Mux/28  "<EngineRhFuelCut>"
  BusSelector/29 -> Mux/29  "<NWCastoring>"
  BusSelector/30 -> Mux/30  "<REFSI_FD_IN_nmodeNoseGearCmd_Deg>"
  BusSelector/31 -> Mux/31  "<REFSI_FD_IN_nmodeSplrLhOutbdCmd_Deg>"
  BusSelector/32 -> Mux/32  "<REFSI_FD_IN_nmodeSplrLhInbdCmd_Deg>"
  BusSelector/33 -> Mux/33  "<REFSI_FD_IN_nmodeSplrRhInbdCmd_Deg>"
  BusSelector/34 -> Mux/34  "<REFSI_FD_IN_nmodeSplrRhOutbdCmd_Deg>"
  BusSelector/35 -> Mux/35  "<REFSI_FD_IN_nmodeCgShifterCmd_Ft>"
  BusSelector/36 -> Mux/36  "<piccoloInCmd>"
  BusSelector/37 -> Mux/37  "<pilotNzCmd_g>"
  BusSelector/38 -> Mux/38  "<isControlSurfaceCmdFromSystem>"
  BusSelector/39 -> Mux/39  "<nmodeReset>"
  BusSelector/40 -> Mux/40  "<RefWindDirDeg>"
  BusSelector/41 -> Mux/41  "<RefWindSpdKts>"
  BusSelector/42 -> Mux/42  "<VertWindSpdKts>"
  BusSelector/43 -> Mux/43  "<PedalBrakeLh>"
  BusSelector/44 -> Mux/44  "<PedalBrakeRh>"
  BusSelector/45 -> Mux/45  "<REFSI_FD_IN_nmodeCgShifterCmd_Flag>"
  BusSelector/46 -> Mux/46  "<REFSI_FD_IN_nmodeCgShifterNRCActive>"

== system Sim_Runs_16p5/DLLSimulation/Vector to Bus ==
  In1 : Inport
  BusCreator : BusCreator  Inputs=149
  Demux : Demux  Outputs=149
  Out1 : Outport
  wires:
  In1/1 -> Demux/1
  BusCreator/1 -> Out1/1
  Demux/1 -> BusCreator/1  "PresAltFt"
  Demux/2 -> BusCreator/2  "AlphaDeg"
  Demux/3 -> BusCreator/3  "BetaDeg"
  Demux/4 -> BusCreator/4  "GammaDeg"
  Demux/5 -> BusCreator/5  "CASKts"
  Demux/6 -> BusCreator/6  "PDps"
  Demux/7 -> BusCreator/7  "QDps"
  Demux/8 -> BusCreator/8  "RDps"
  Demux/9 -> BusCreator/9  "PhiDeg"
  Demux/10 -> BusCreator/10  "ThetaDeg"
  Demux/11 -> BusCreator/11  "PsiDeg"
  Demux/12 -> BusCreator/12  "TASKts"
  Demux/13 -> BusCreator/13  "HeightAGLFt"
  Demux/14 -> BusCreator/14  "XthrustLbs"
  Demux/15 -> BusCreator/15  "GrndContactLMG"
  Demux/16 -> BusCreator/16  "GrndContactNG"
  Demux/17 -> BusCreator/17  "GrndContactRMG"
  Demux/18 -> BusCreator/18  "DynPresPsf"
  Demux/19 -> BusCreator/19  "PAmbPsf"
  Demux/20 -> BusCreator/20  "XposnFt"
  Demux/21 -> BusCreator/21  "YposnFt"
  Demux/22 -> BusCreator/22  "ZposnFt"
  Demux/23 -> BusCreator/23  "NxG"
  Demux/24 -> BusCreator/24  "NyG"
  Demux/25 -> BusCreator/25  "NzG"
  Demux/26 -> BusCreator/26  "VEarthFtps_0"
  Demux/27 -> BusCreator/27  "VEarthFtps_1"
  Demux/28 -> BusCreator/28  "VEarthFtps_2"
  Demux/29 -> BusCreator/29  "LatitudeDeg"
  Demux/30 -> BusCreator/30  "LongitudeDeg"
  Demux/31 -> BusCreator/31  "ZgrndLhLbs"
  Demux/32 -> BusCreator/32  "ZgrndRhLbs"
  Demux/33 -> BusCreator/33  "ZgrndNgLbs"
  Demux/34 -> BusCreator/34  "Time"
  Demux/35 -> BusCreator/35  "WindUFtps"
  Demux/36 -> BusCreator/36  "WindVFtps"
  Demux/37 -> BusCreator/37  "WindWFtps"
  Demux/38 -> BusCreator/38  "AilLwrLhBDriveDeg"
  Demux/39 -> BusCreator/39  "AilUprLhBDriveDeg"
  Demux/40 -> BusCreator/40  "AilLwrRhBDriveDeg"
  Demux/41 -> BusCreator/41  "AilUprRhBDriveDeg"
  Demux/42 -> BusCreator/42  "ElvLhOBBDriveDeg"
  Demux/43 -> BusCreator/43  "ElvLhIBBDriveDeg"
  Demux/44 -> BusCreator/44  "ElvRhOBBDriveDeg"
  Demux/45 -> BusCreator/45  "ElvRhIBBDriveDeg"
  Demux/46 -> BusCreator/46  "RudPylLhBDriveDeg"
  Demux/47 -> BusCreator/47  "RudUTailLhBDriveDeg"
  Demux/48 -> BusCreator/48  "RudWingletLhBDriveDeg"
  Demux/49 -> BusCreator/49  "ElvUTailLhBDriveDeg"
  Demux/50 -> BusCreator/50  "ElvUTailRhBDriveDeg"
  Demux/51 -> BusCreator/51  "RudPylRhBDriveDeg"
  Demux/52 -> BusCreator/52  "RudUTailRhBDriveDeg"
  Demux/53 -> BusCreator/53  "RudWingletRhBDriveDeg"
  Demux/54 -> BusCreator/54  "AftFlapBDriveDeg"
  Demux/55 -> BusCreator/55  "NWBDriveDeg"
  Demux/56 -> BusCreator/56  "XcgPctMAC"
  Demux/57 -> BusCreator/57  "IxxLbsInch2"
  Demux/58 -> BusCreator/58  "IyyLbsInch2"
  Demux/59 -> BusCreator/59  "IzzLbsInch2"
  Demux/60 -> BusCreator/60  "IxzLbsInch2"
  Demux/61 -> BusCreator/61  "REFSI_FD_OUT_PIC_dynPres_Pa"
  Demux/62 -> BusCreator/62  "REFSI_FD_OUT_PIC_TAmb_C"
  Demux/63 -> BusCreator/63  "REFSI_FD_OUT_PIC_PAmb_Pa"
  Demux/64 -> BusCreator/64  "REFSI_FD_OUT_PIC_rollRate_Dps"
  Demux/65 -> BusCreator/65  "REFSI_FD_OUT_PIC_pitchRate_Dps"
  Demux/66 -> BusCreator/66  "REFSI_FD_OUT_PIC_yawRate_Dps"
  Demux/67 -> BusCreator/67  "REFSI_FD_OUT_PIC_accelXDir_Mps2"
  Demux/68 -> BusCreator/68  "REFSI_FD_OUT_PIC_accelYDir_Mps2"
  Demux/69 -> BusCreator/69  "REFSI_FD_OUT_PIC_accelZDir_Mps2"
  Demux/70 -> BusCreator/70  "REFSI_FD_OUT_PIC_GPSUbloxLatitudeDeg"
  Demux/71 -> BusCreator/71  "REFSI_FD_OUT_PIC_GPSUbloxLongitudeDeg"
  Demux/72 -> BusCreator/72  "REFSI_FD_OUT_PIC_GPSUbloxHeight_m"
  Demux/73 -> BusCreator/73  "REFSI_FD_OUT_PIC_vEarthXUblox_Mps"
  Demux/74 -> BusCreator/74  "REFSI_FD_OUT_PIC_vEarthYUblox_Mps"
  Demux/75 -> BusCreator/75  "REFSI_FD_OUT_PIC_vEarthZUblox_Mps"
  Demux/76 -> BusCreator/76  "REFSI_FD_OUT_PIC_GPSNovAftLatitudeDeg"
  Demux/77 -> BusCreator/77  "REFSI_FD_OUT_PIC_GPSNovAftLongitudeDeg"
  Demux/78 -> BusCreator/78  "REFSI_FD_OUT_PIC_GPSNovAftHeight_m"
  Demux/79 -> BusCreator/79  "REFSI_FD_OUT_PIC_vEarthXNovAft_Mps"
  Demux/80 -> BusCreator/80  "REFSI_FD_OUT_PIC_vEarthYNovAft_Mps"
  Demux/81 -> BusCreator/81  "REFSI_FD_OUT_PIC_vEarthZNovAft_Mps"
  Demux/82 -> BusCreator/82  "ismCas_Kt"
  Demux/83 -> BusCreator/83  "ismTas_Kt"
  Demux/84 -> BusCreator/84  "ismPresAlt_Ft"
  Demux/85 -> BusCreator/85  "ismDynPres_Psf"
  Demux/86 -> BusCreator/86  "ismAoa_Deg"
  Demux/87 -> BusCreator/87  "ismAos_Deg"
  Demux/88 -> BusCreator/88  "speedIncrementImuXRaw_Mps"
  Demux/89 -> BusCreator/89  "speedIncrementImuYRaw_Mps"
  Demux/90 -> BusCreator/90  "speedIncrementImuZRaw_Mps"
  Demux/91 -> BusCreator/91  "rollIncrementRaw_Deg"
  Demux/92 -> BusCreator/92  "pitchIncrementRaw_Deg"
  Demux/93 -> BusCreator/93  "yawIncrementRaw_Deg"
  Demux/94 -> BusCreator/94  "latitudeRaw_Rad"
  Demux/95 -> BusCreator/95  "longitudeRaw_Rad"
  Demux/96 -> BusCreator/96  "heightRaw_M"
  Demux/97 -> BusCreator/97  "speedGpsIneNavXRaw_Mps"
  Demux/98 -> BusCreator/98  "speedGpsIneNavYRaw_Mps"
  Demux/99 -> BusCreator/99  "speedGpsIneNavZRaw_Mps"
  Demux/100 -> BusCreator/100  "isGpsMeasurementValid"
  Demux/101 -> BusCreator/101  "gpsDelay_s"
  Demux/102 -> BusCreator/102  "latitudeStandardDeviation_M"
  Demux/103 -> BusCreator/103  "longitudeStandardDeviation_M"
  Demux/104 -> BusCreator/104  "heightStandardDeviation_M"
  Demux/105 -> BusCreator/105  "speedXStandardDeviation_Mps"
  Demux/106 -> BusCreator/106  "speedYStandardDeviation_Mps"
  Demux/107 -> BusCreator/107  "speedZStandardDeviation_Mps"
  Demux/108 -> BusCreator/108  "gpsMode"
  Demux/109 -> BusCreator/109  "latitudePiccolo_Rad"
  Demux/110 -> BusCreator/110  "longitudePiccolo_Rad"
  Demux/111 -> BusCreator/111  "heightPiccolo_M"
  Demux/112 -> BusCreator/112  "speedGpsIneNavXPiccolo_Mps"
  Demux/113 -> BusCreator/113  "speedGpsIneNavYPiccolo_Mps"
  Demux/114 -> BusCreator/114  "speedGpsIneNavZPiccolo_Mps"
  Demux/115 -> BusCreator/115  "rollAttitudePiccolo_Deg"
  Demux/116 -> BusCreator/116  "pitchAttitudePiccolo_Deg"
  Demux/117 -> BusCreator/117  "yawAttitudePiccolo_Deg"
  Demux/118 -> BusCreator/118  "rollRatePiccolo_Dps"
  Demux/119 -> BusCreator/119  "pitchRatePiccolo_Dps"
  Demux/120 -> BusCreator/120  "yawRatePiccolo_Dps"
  Demux/121 -> BusCreator/121  "nxPiccolo"
  Demux/122 -> BusCreator/122  "nyPiccolo"
  Demux/123 -> BusCreator/123  "nzPiccolo"
  Demux/124 -> BusCreator/124  "piccoloDelay_s"
  Demux/125 -> BusCreator/125  "ismTLALh_Deg"
  Demux/126 -> BusCreator/126  "ismTLARh_Deg"
  Demux/127 -> BusCreator/127  "REFSI_AC_OUT_nmodeRudLhWingCmd_Deg"
  Demux/128 -> BusCreator/128  "REFSI_AC_OUT_nmodeAilLhLowerCmd_Deg"
  Demux/129 -> BusCreator/129  "REFSI_AC_OUT_nmodeAilLhUpperCmd_Deg"
  Demux/130 -> BusCreator/130  "REFSI_AC_OUT_nmodeElvLhOutbdCmd_Deg"
  Demux/131 -> BusCreator/131  "REFSI_AC_OUT_nmodeElvLhInbdCmd_Deg"
  Demux/132 -> BusCreator/132  "REFSI_AC_OUT_nmodeRudLhPylonCmd_Deg"
  Demux/133 -> BusCreator/133  "REFSI_AC_OUT_nmodeRudLhUTailCmd_Deg"
  Demux/134 -> BusCreator/134  "REFSI_AC_OUT_nmodeElvLhUTailCmd_Deg"
  Demux/135 -> BusCreator/135  "REFSI_AC_OUT_nmodeAftFlapCmd_Deg"
  Demux/136 -> BusCreator/136  "REFSI_AC_OUT_nmodeElvRhUTailCmd_Deg"
  Demux/137 -> BusCreator/137  "REFSI_AC_OUT_nmodeRudRhUTailCmd_Deg"
  Demux/138 -> BusCreator/138  "REFSI_AC_OUT_nmodeRudRhPylonCmd_Deg"
  Demux/139 -> BusCreator/139  "REFSI_AC_OUT_nmodeElvRhInbdCmd_Deg"
  Demux/140 -> BusCreator/140  "REFSI_AC_OUT_nmodeElvRhOutbdCmd_Deg"
  Demux/141 -> BusCreator/141  "REFSI_AC_OUT_nmodeAilRhUpperCmd_Deg"
  Demux/142 -> BusCreator/142  "REFSI_AC_OUT_nmodeAilRhLowerCmd_Deg"
  Demux/143 -> BusCreator/143  "REFSI_AC_OUT_nmodeRudRhWingCmd_Deg"
  Demux/144 -> BusCreator/144  "VoltageLhEngine"
  Demux/145 -> BusCreator/145  "VoltageRhEngine"
  Demux/146 -> BusCreator/146  "VoltagePWMLhEngine"
  Demux/147 -> BusCreator/147  "VoltagePWMRhEngine"
  Demux/148 -> BusCreator/148  "CurrentLhEngine"
  Demux/149 -> BusCreator/149  "CurrentRhEngine"
